simulink model "robot_capteur_etu"  (R2019a)
settings: Solver=VariableStepAuto  StartTime=0.0  StopTime=10.0  RelTol=1e-3
values from neighbouring files (symbols this model uses):
  K = -place(A,B,poles)    [matrices.m]    (also in simu_robot_etu.m = [0 0 0 0]; simulation_robot.m = K_tab(i,:))
  ue = 0    [simu_robot_etu.m]
  x0 = [0 0 0 0]'    [simu_robot_etu.m]    (also in simulation_robot.m = [0 pi/4 0 0]')
  xe = [0 0 0 0]'    [simu_robot_etu.m]
settings Model: Creator=nfoin  LastModifiedBy=nfoin

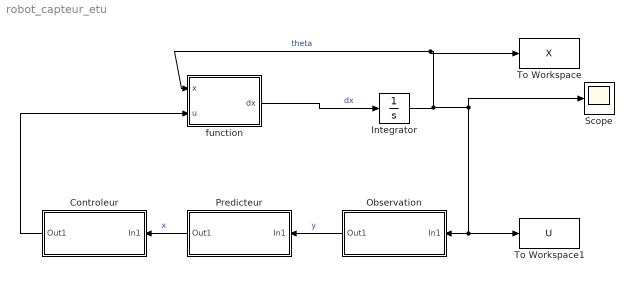
== system robot_capteur_etu ==
  Controleur : Subsystem
  Integrator : Integrator  InitialCondition=x0
  Observation : Subsystem
  Predicteur : Subsystem
  Scope : Scope
  To Workspace : ToWorkspace  VariableName=X  SaveFormat=Timeseries  SampleTime=-1
  To Workspace1 : ToWorkspace  VariableName=U  SaveFormat=Timeseries  SampleTime=-1
  function : MATLAB Function  TreatAsAtomicUnit=on
  wires:
  function/1(dx) -> Integrator/1  "dx"
  Observation/1(Out1) -> Predicteur/1(In1)  "y"
  Predicteur/1(Out1) -> Controleur/1(In1)  "x"
  Controleur/1(Out1) -> function/2(u)
  Integrator/1 -> To Workspace/1, function/1(x), To Workspace1/1, Observation/1(In1), Scope/1  "theta"

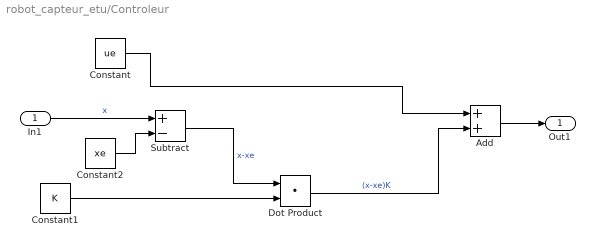
== system robot_capteur_etu/Controleur ==
  In1 : Inport
  Add : Sum
  Constant : Constant  Value=ue
  Constant1 : Constant  Value=K
  Constant2 : Constant  Value=xe
  Dot Product : DotProduct  InputSameDT=on  OutDataTypeStr=Inherit: Inherit via internal rule
  Subtract : Sum  Inputs=+-
  Out1 : Outport
  wires:
  In1/1 -> Subtract/1  "x"
  Constant/1 -> Add/1
  Constant1/1 -> Dot Product/2
  Constant2/1 -> Subtract/2
  Subtract/1 -> Dot Product/1  "x-xe"
  Dot Product/1 -> Add/2  "(x-xe)K"
  Add/1 -> Out1/1

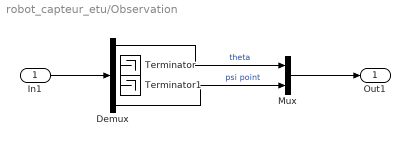
== system robot_capteur_etu/Observation ==
  In1 : Inport
  Demux : Demux
  Mux : Mux  Inputs=2
  Terminator : Terminator
  Terminator1 : Terminator
  Out1 : Outport
  wires:
  In1/1 -> Demux/1
  Mux/1 -> Out1/1
  Demux/1 -> Mux/1  "theta"
  Demux/4 -> Mux/2  "psi point"

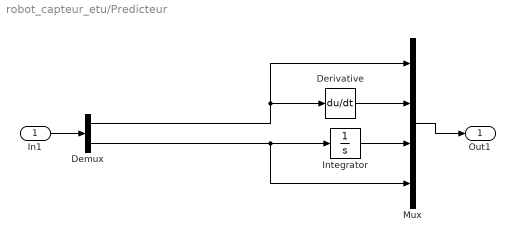
== system robot_capteur_etu/Predicteur ==
  In1 : Inport
  Demux : Demux  Outputs=2
  Derivative : Derivative
  Integrator : Integrator
  Mux : Mux
  Out1 : Outport
  wires:
  In1/1 -> Demux/1
  Mux/1 -> Out1/1
  Demux/1 -> Derivative/1, Mux/1
  Demux/2 -> Integrator/1, Mux/4
  Integrator/1 -> Mux/3
  Derivative/1 -> Mux/2

== matlab function robot_capteur_etu/function ==
  data: x input; u input; dx output
function dx   = fcn( x, u)
%   Dynamic equations of motion of the segway on an axis.
%   Inputs: - x = [theta psi dtheta dpsi]
%               theta: average angle of the wheels      [rad]
%               psi: body pitch angle                   [rad]
%               dtheta: average velocity of the wheels  [rad/s]
%               dpsi: body pitch velocity               [rad/s]
%          - u: DC motor voltage (same value for both motors) [V]

    % State
    size(x)
    psi = x(2);
    dtheta = x(3);
    dpsi = x(4);

    % Parameters
    
    g = 9.81;           % gravity acceleration [m/sec^2]
    m = 0.03;           % wheel weight [kg]
    R = 0.04;           % wheel radius [m]
    Jw = m*R^2/2;       % wheel inertia moment [kg*m^2]
    M = 0.6;            % body weight [kg]
    H = 0.144;          % body height [m]
    L = H/2;            % distance of the center of mass from the wheel axle [m]
    Jpsi = M*L^2/3;     % body pitch inertia [kgm^2]
    Jm = 1e-5;          % DC motor inertia moment [kgm^2]
    Rm = 6.69;          % DC motor resistance [Ohm]
    Kb = 0.468;         % DC motor back EMF constant [Vsec/rad]
    Kt = 0.317;         % DC motor torque constant [Nm/A]
    n = 1;              % gear ratio
    fm = 0.0022;        % friction coefficient between body and DC motor
    fw = 0;             % friction coefficient between wheel and floor
    
    % Equations of motion
    c1 = (2*m+M)*R^2 + 2*Jw + 2*n^2*Jm;
    c2 = M*L*R*cos(psi) - 2*n^2*Jm;
    c3 = -M*L*R*dpsi^2*sin(psi);
    c4 = M*L^2 + Jpsi + 2*n^2*Jm;
    c5 = -M*g*L*sin(psi);

    alpha = Kt/Rm;
    beta = Kt*Kb/Rm + fm;

    Ftheta = alpha*(2*u) - 2*(beta+fw)*dtheta + 2*beta*dpsi;
    Fpsi = -alpha*(2*u) + 2*beta*dtheta - 2*beta*dpsi;

    ddtheta = (c4*c3 - c2*c5 + c4*Ftheta - c2*Fpsi)/(c4*c1 - c2^2);
    ddpsi = (Fpsi- c2*ddtheta - c5)/c4;
    dx = [dtheta dpsi ddtheta ddpsi]';

end
